simulink subsystem "Multibody_Input_Calibration"  (R2022b)
settings: Solver=VariableStepAuto  StartTime=0.0  StopTime=10.0  RelTol=1e-3
settings Model: Creator=david  LastModifiedBy=david

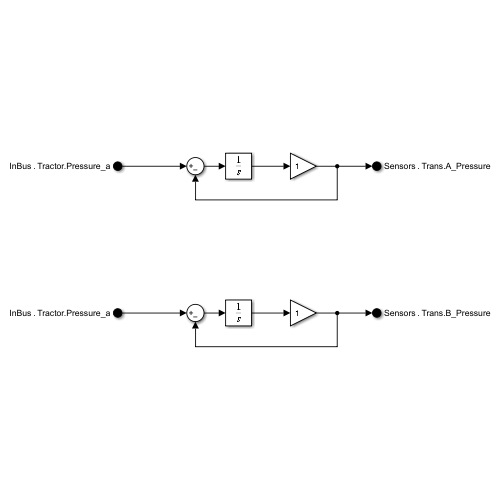
[thumbnail: Simulink's stored preview of the top-level diagram]
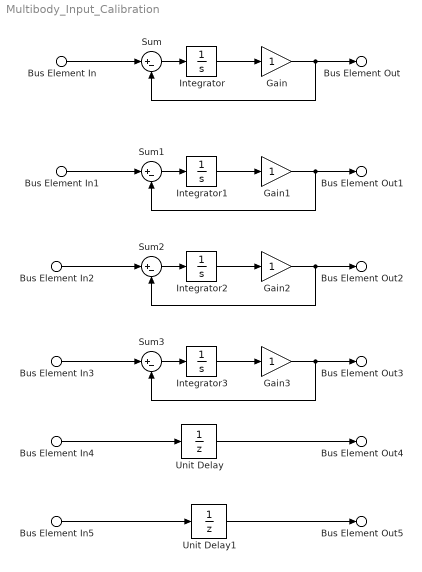
== system Multibody_Input_Calibration ==
  Bus Element In : Inport  PortName=InBus  Element=Tractor.Pressure_A
  Bus Element In1 : Inport  PortName=InBus  Element=Tractor.Pressure_B
  Bus Element In2 : Inport  PortName=InBus  Element=Tractor.MP1_Speed
  Bus Element In3 : Inport  PortName=InBus  Element=Tractor.MP2_Speed
  Bus Element In4 : Inport  PortName=InBus  Element=Tractor.MP1_Swash
  Bus Element In5 : Inport  PortName=InBus  Element=Tractor.MP2_Swash
  Gain{,1..3} (4 alike) : Gain
  Integrator{,1..3} (4 alike) : Integrator
  Sum{,1..3} (4 alike) : Sum  Inputs=|+-
  Unit Delay : UnitDelay  SampleTime=-1  HasFrameUpgradeWarning=on
  Unit Delay1 : UnitDelay  SampleTime=-1  HasFrameUpgradeWarning=on
  Bus Element Out : Outport  VectorParamsAs1DForOutWhenUnconnected=off  PortName=Sensors  Element=Trans.Pressure_A
  Bus Element Out1 : Outport  VectorParamsAs1DForOutWhenUnconnected=off  PortName=Sensors  Element=Trans.Pressure_B
  Bus Element Out2 : Outport  VectorParamsAs1DForOutWhenUnconnected=off  PortName=Sensors  Element=Trans.MP1_Speed
  Bus Element Out3 : Outport  VectorParamsAs1DForOutWhenUnconnected=off  PortName=Sensors  Element=Trans.MP2_Speed
  Bus Element Out4 : Outport  VectorParamsAs1DForOutWhenUnconnected=off  PortName=Sensors  Element=Trans.MP1_Swash
  Bus Element Out5 : Outport  VectorParamsAs1DForOutWhenUnconnected=off  PortName=Sensors  Element=Trans.MP2_Swash
  wires:
  Sum/1 -> Integrator/1
  Integrator/1 -> Gain/1
  Gain/1 -> Bus Element Out/1, Sum/2
  Bus Element In/1 -> Sum/1
  Bus Element In1/1 -> Sum1/1
  Gain1/1 -> Bus Element Out1/1, Sum1/2
  Integrator1/1 -> Gain1/1
  Sum1/1 -> Integrator1/1
  Sum2/1 -> Integrator2/1
  Integrator2/1 -> Gain2/1
  Gain2/1 -> Sum2/2, Bus Element Out2/1
  Bus Element In2/1 -> Sum2/1
  Bus Element In3/1 -> Sum3/1
  Gain3/1 -> Sum3/2, Bus Element Out3/1
  Integrator3/1 -> Gain3/1
  Sum3/1 -> Integrator3/1
  Bus Element In4/1 -> Unit Delay/1
  Unit Delay/1 -> Bus Element Out4/1
  Bus Element In5/1 -> Unit Delay1/1
  Unit Delay1/1 -> Bus Element Out5/1
